simulink model "scheme2"  (R2014a)
settings: Solver=ode45  StartTime=0.0  StopTime=1  MaxStep=0.001  MinStep=0.0001  RelTol=1e-3
libraries: simulink x1
settings Model: Creator=User  LastModifiedBy=Анастасия

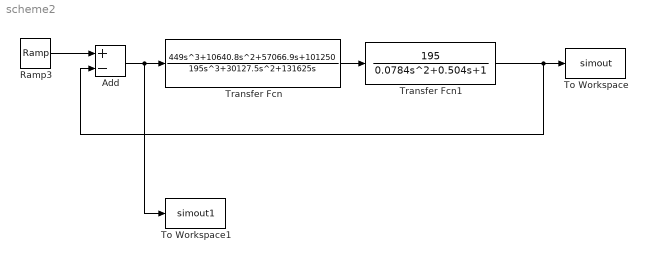
== system scheme2 ==
  Add : Sum  Inputs=+-
  Ramp3 : simulink/Sources/Ramp  slope=6  start=0  X0=0
  To Workspace : ToWorkspace  VariableName=simout  SaveFormat=Timeseries  SampleTime=-1
  To Workspace1 : ToWorkspace  VariableName=simout1  SaveFormat=Timeseries  SampleTime=-1
  Transfer Fcn : TransferFcn  Numerator=[449 10640.8 57066.9 101250]  Denominator=[195 30127.5 131625 0]
  Transfer Fcn1 : TransferFcn  Numerator=[195]  Denominator=[0.0784 0.504 1 ]
  wires:
  Add/1 -> To Workspace1/1, Transfer Fcn/1
  Transfer Fcn/1 -> Transfer Fcn1/1
  Ramp3/1 -> Add/1
  Transfer Fcn1/1 -> Add/2, To Workspace/1
